simulink subsystem "TOAD_TrajectoryGen_2"  (R2025a)
settings: Solver=VariableStepAuto  StartTime=0.0  StopTime=10.0  RelTol=1e-3
settings Model: Creator=pplat  LastModifiedBy=pplata

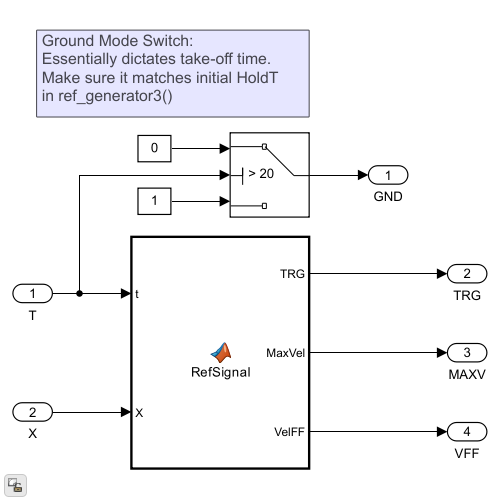
[thumbnail: Simulink's stored preview of the top-level diagram]
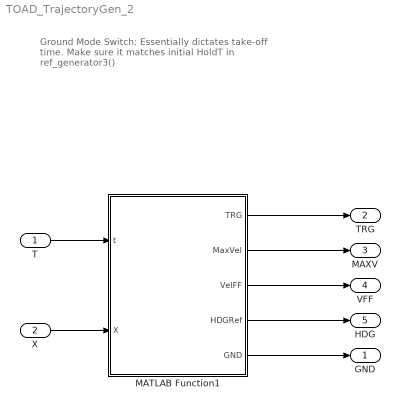
== system TOAD_TrajectoryGen_2 ==
  note: Ground Mode Switch:
      | Essentially dictates take-off time.
      | Make sure it matches initial HoldT
      | in ref_generator3()
  T : Inport
  X : Inport  Port=2  PortDimensions=[15,1]
  MATLAB Function1 : MATLAB Function  TreatAsAtomicUnit=on
  GND : Outport
  TRG : Outport  Port=2
  MAXV : Outport  Port=3
  VFF : Outport  Port=4
  HDG : Outport  Port=5
  wires:
  MATLAB Function1/2(MaxVel) -> MAXV/1
  MATLAB Function1/3(VelFF) -> VFF/1
  X/1 -> MATLAB Function1/2(X)
  MATLAB Function1/1(TRG) -> TRG/1
  T/1 -> MATLAB Function1/1(t)
  MATLAB Function1/4(HDGRef) -> HDG/1
  MATLAB Function1/5(GND) -> GND/1

== matlab function TOAD_TrajectoryGen_2/MATLAB Function1 ==
  data: t input; X input; TRG output; MaxVel output; VelFF output; HDGRef output; GND output
function [TRG, MaxVel, VelFF, HDGRef, GND] = RefSignal(t, X)

[TRG, MaxVel, VelFF, HDGRef, GND] = WaypointCommands(X, t);
